simulink model "QuarterCar_FLC"  (R2014a)
settings: Solver=ode4  StartTime=0.0  StopTime=5  FixedStep=0.001  RelTol=1e-3
undefined symbols (not defined in the file): A1, A2, w_vec
libraries: fuzblock x1
settings Model: Creator=MLRida  LastModifiedBy=MLRida

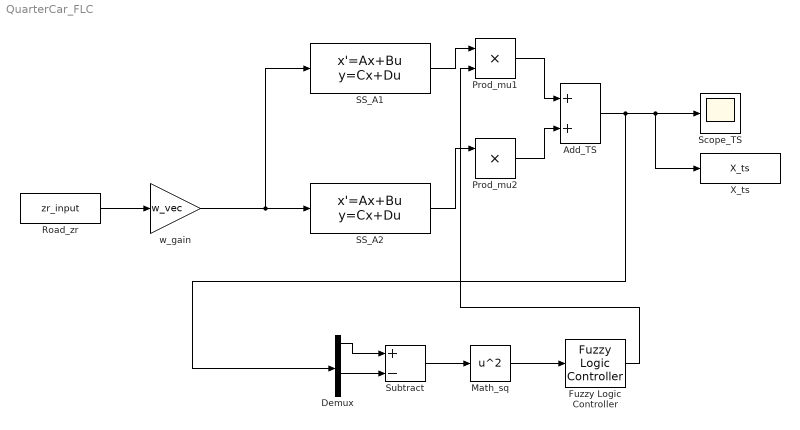
== system QuarterCar_FLC ==
  Add_TS : Sum
  Demux : Demux
  Fuzzy Logic Controller : fuzblock/Fuzzy Logic  Controller  fis=TS_model
  Math_sq : Math  Operator=square  SaturateOnIntegerOverflow=on
  Prod_mu1 : Product
  Prod_mu2 : Product
  Road_zr : FromWorkspace  VariableName=zr_input  SampleTime=0.001
  SS_A1 : StateSpace  A=A1  B=eye(4)  C=eye(4)  D=zeros(4,4)  X0=[0;0;0;0]
  SS_A2 : StateSpace  A=A2  B=eye(4)  C=eye(4)  D=zeros(4,4)  X0=[0;0;0;0]
  Scope_TS : Scope
  Subtract : Sum  Inputs=+-
  X_ts : ToWorkspace  VariableName=X_ts  SampleTime=-1
  w_gain : Gain  Gain=w_vec
  wires:
  Road_zr/1 -> w_gain/1
  w_gain/1 -> SS_A1/1, SS_A2/1
  SS_A1/1 -> Prod_mu1/1
  SS_A2/1 -> Prod_mu2/1
  Prod_mu1/1 -> Add_TS/1
  Prod_mu2/1 -> Add_TS/2
  Add_TS/1 -> Scope_TS/1, X_ts/1, Demux/1
  Demux/1 -> Subtract/1
  Demux/3 -> Subtract/2
  Subtract/1 -> Math_sq/1
  Math_sq/1 -> Fuzzy Logic Controller/1
  Fuzzy Logic Controller/1 -> Prod_mu1/2
